simulink model "bergman_GA"  (R2021a)
settings: Solver=FixedStepAuto  StartTime=0.0  StopTime=time(end)  FixedStep=1e-2  RelTol=1e-3
values from neighbouring files (symbols this model uses):
  G_0 = 14.9    [cv3.m]    (also in cv3a.m = 13.5; gaResults.m = Best(4); tuneGA.m = pop(i,4))
  Gb = 153    [afterGA.m]    (also in bergmanGA.m = glucose(1); cv3.m = glucose(1); cv3a.m = glucose(1); cv4_bergman.m)
  glucose = ar(:,2)    [bergmanGA.m]    (also in cv3.m; cv3a.m; gaResults.m)
  Ib = 12.3165    [afterGA.m]    (also in bergmanGA.m = insuline(1); cv3.m = insuline(1); cv3a.m = insuline(1); cv4.m)
  insuline = ar(:,3)    [bergmanGA.m]    (also in cv3.m; cv3a.m; gaResults.m)
  p2 = 0.0106    [afterGA.m]    (also in cv3.m = 0.032736; cv3a.m = 0.063098; cv4_bergman.m = Best(2) / 10; cv4_bergmanGA.m = Best(2) / 10)
  Sg = 0.032    [afterGA.m]    (also in cv3.m = 0.030031; cv3a.m = 3.3574e-10; cv4_bergman.m = 0; cv4_bergmanGA.m = 0)
  Si = 0.00159    [afterGA.m]    (also in cv3.m = 1.0278e-13; cv3a.m = 0.00089844; cv4_bergman.m = Best(1) / 10; cv4_bergmanGA.m = Best(1) / 10)
  time = ar(:,1)    [bergmanGA.m]    (also in cv3.m; cv3a.m; gaResults.m; surove.m = s1.time)
settings Model: Creator=marko  LastModifiedBy=marko

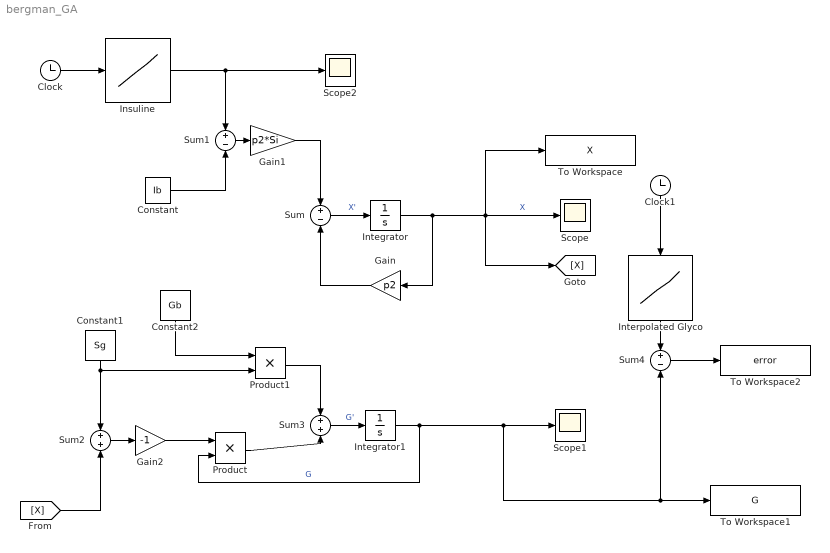
== system bergman_GA ==
  Clock : Clock
  Clock1 : Clock
  Constant : Constant  Value=Ib
  Constant1 : Constant  Value=Sg
  Constant2 : Constant  Value=Gb
  Gain : Gain  Gain=p2
  Gain1 : Gain  Gain=p2*Si
  Gain2 : Gain  Gain=-1
  Insuline : Lookup_n-D  NumberOfTableDimensions=1  BreakpointsForDimension1=time  Table=insuline  InternalRulePriority=Speed  RndMeth=Simplest  InputSameDT=on
  Integrator : Integrator
  Integrator1 : Integrator  InitialCondition=G_0
  Interpolated Glyco : Lookup_n-D  NumberOfTableDimensions=1  BreakpointsForDimension1=time  Table=glucose  InternalRulePriority=Speed  RndMeth=Simplest  InputSameDT=on
  Product : Product
  Product1 : Product
  Scope : Scope
  Scope1 : Scope
  Scope2 : Scope
  Sum : Sum  Inputs=+|-
  Sum1 : Sum  Inputs=+|-
  Sum2 : Sum
  Sum3 : Sum
  Sum4 : Sum  Inputs=+|-
  To Workspace : ToWorkspace  VariableName=X  SaveFormat=Timeseries  SampleTime=-1
  To Workspace1 : ToWorkspace  VariableName=G  SaveFormat=Timeseries  SampleTime=-1
  To Workspace2 : ToWorkspace  VariableName=error  SampleTime=-1
  wires:
  Integrator/1 -> To Workspace/1, [X], Scope/1, Gain/1  "X"
  Gain/1 -> Sum/2
  Sum/1 -> Integrator/1  "X'"
  Clock/1 -> Insuline/1
  Constant/1 -> Sum1/2
  Insuline/1 -> Sum1/1, Scope2/1
  Sum1/1 -> Gain1/1
  Gain1/1 -> Sum/1
  Sum2/1 -> Gain2/1
  Gain2/1 -> Product/1
  Integrator1/1 -> Sum4/2, To Workspace1/1, Scope1/1, Product/2  "G"
  Constant1/1 -> Sum2/1, Product1/2
  [X] -> Sum2/2
  Product/1 -> Sum3/2
  Product1/1 -> Sum3/1
  Constant2/1 -> Product1/1
  Sum3/1 -> Integrator1/1  "G'"
  Clock1/1 -> Interpolated Glyco/1
  Interpolated Glyco/1 -> Sum4/1
  Sum4/1 -> To Workspace2/1
